simulink model "Water_Tank_Plant_Model"  (R2022b)
settings: Solver=VariableStepAuto  StartTime=0.0  StopTime=inf  RelTol=1e-3
model workspace (MAT data in the model file):
  A = 8
  Boost = 0
  Empty = 0
  Height = 3
  Hin = 8
  Qin = 2
  R = 1
  b = 0
libraries: slpidlib x1
settings Model: Creator=deanlonergan  LastModifiedBy=deanlonergan

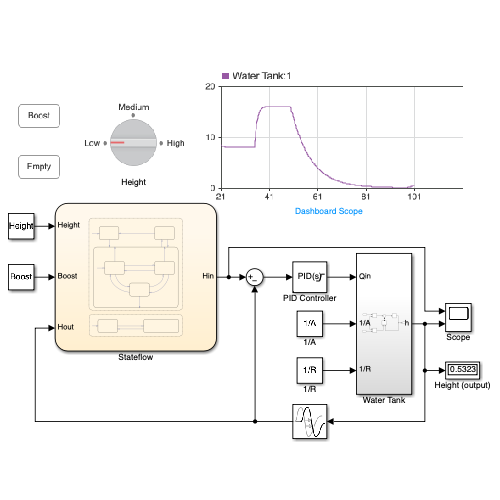
[thumbnail: Simulink's stored preview of the top-level diagram]
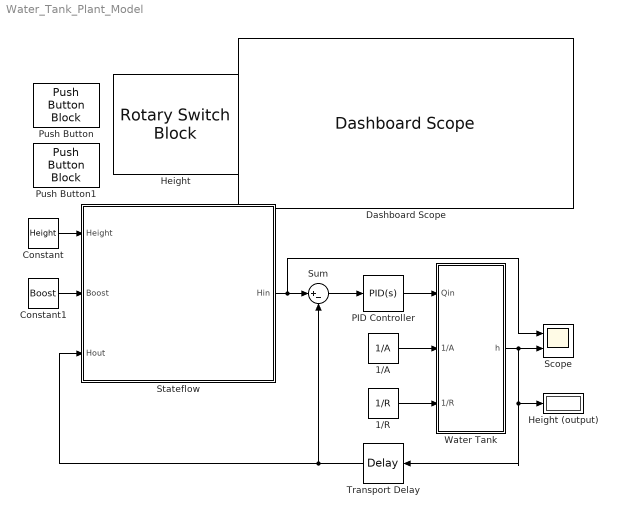
== system Water_Tank_Plant_Model ==
  1/A : Constant  Value=1/A
  1/R : Constant  Value=1/R
  Constant : Constant  Value=Height
  Constant1 : Constant  Value=Boost
  Dashboard Scope : DashboardScope  Ymin=0  Ymax=20  ScaleAtStop=off  UpdateMode=Scroll
  Height : RotarySwitchBlock  LabelPosition=Hide
      settings: Values={{'Low', 'Medium', 'High'}, [1 2 3]}
  Height (output) : Display
  PID Controller : slpidlib/PID Controller  Controller=PID  Form=Parallel  TimeDomain=Continuous-time  UseExternalTs=off  SampleTime=-1  IntegratorMethod=Forward Euler  FilterMethod=Forward Euler  ControllerParametersSource=internal  P=7.2  I=0.92  UseKiTs=on  D=0.29  N=0  UseFilter=on  TunerSelectOption=Transfer Function Based (PID Tuner App)  InitialConditionSource=internal  InitialConditionForIntegrator=0  InitialConditionForFilter=0  DifferentiatorICPrevScaledInput=0  ExternalReset=none  TrackingMode=off  Kt=1  LimitOutput=on  SatLimitsSource=internal  UpperSaturationLimit=50  LowerSaturationLimit=-0  LinearizeAsGain=on  AntiWindupMode=none  Kb=1  LimitIntegrator=off  UpperIntegratorSaturationLimit=inf  LowerIntegratorSaturationLimit=-inf  POutMin=[]  POutMax=[]  IOutMin=[]  IOutMax=[]  DOutMin=[]  DOutMax=[]  NOutMin=[]  NOutMax=[]  SumOutMin=[]  SumOutMax=[]  SaturationOutMin=[]  SaturationOutMax=[]  PParamMin=[]  PParamMax=[]  IParamMin=[]  IParamMax=[]  DParamMin=[]  DParamMax=[]  NParamMin=[]  NParamMax=[]  KbParamMin=[]  KbParamMax=[]  KtParamMin=[]  KtParamMax=[]  KbOutMin=[]  KbOutMax=[]  KtOutMin=[]  KtOutMax=[]  IntegratorOutMin=[]  IntegratorOutMax=[]  FilterOutMin=[]  FilterOutMax=[]  SumI1OutMin=[]  SumI1OutMax=[]  SumI2OutMin=[]  SumI2OutMax=[]  SumI3OutMin=[]  SumI3OutMax=[]  SumI4OutMin=[]  SumI4OutMax=[]  SumDOutMin=[]  SumDOutMax=[]  DifferentiatorOutMin=[]  DifferentiatorOutMax=[]  FilterDiffOutCoefMin=[]  FilterDiffOutCoefMax=[]  ReciprocalOutMin=[]  ReciprocalOutMax=[]  SumDenOutMin=[]  SumDenOutMax=[]  SumNumOutMin=[]  SumNumOutMax=[]  DivideOutMin=[]  DivideOutMax=[]  UdiffTsProdOutMin=[]  UdiffTsProdOutMax=[]  NTsProdOutMin=[]  NTsProdOutMax=[]  UintegralTsProdOutMin=[]  UintegralTsProdOutMax=[]  UngainTsProdOutMin=[]  UngainTsProdOutMax=[]  ClampingZeroOutDataTypeStr=Inherit: Inherit via back propagation  ClampingZeroOutMin=[]  ClampingZeroOutMax=[]  FilterDenConstantOutDataTypeStr=Inherit: Inherit via back propagation  FilterDenConstantOutMin=[]  FilterDenConstantOutMax=[]  PCopyOutDataTypeStr=Inherit: Inherit via back propagation  PCopyOutMin=[]  PCopyOutMax=[]  NCopyOutDataTypeStr=Inherit: Inherit via back propagation  NCopyOutMin=[]  NCopyOutMax=[]  IntegratorContinuousStateAttributes=''  IntegratorStateMustResolveToSignalObject=off  IntegratorRTWStateStorageClass=Auto  FilterContinuousStateAttributes=''  FilterStateMustResolveToSignalObject=off  FilterRTWStateStorageClass=Auto  ParallelPVariant=InternalParameters  IdealPVariant=Disabled  IVariant=InternalParameters  DVariant=InternalParameters  IntegratorVariant=Continuous  SatVariant=Enabled  AWVariant=Passthrough  PCopyVariant=Disabled  TRVariant=Disabled  FdbkBlocksVariant=Forward  IdealPFdbkVariant=Disabled  SatFdbkVariant=Disabled  DerivativeFilterVariant=ContFilter  NVariant=InternalParameters  NCopyVariant=Disabled  FilterICVariant=InternalICsFilter  IntegratorICVariant=InternalICs  ExternalResetVariant=Disabled  TRSumVariant=Passthrough  SumFdbkVariant=Disabled  SumVariant=Sum_PID  TsampFilterVariant=InternalTs  TsampNgainVariant=Passthrough  TsampIntegralVariant=Passthrough  ExternalSaturationOutDataTypeStr=Inherit: Same as second input
  Push Button : PushButtonBlock  ButtonText=Boost  OffValue=0.000000
  Push Button1 : PushButtonBlock  ButtonText=Empty  OnValue=0  OffValue=3.000000
  Scope : Scope  NumInputPorts=2
  Stateflow : Stateflow chart  TreatAsAtomicUnit=on
  Sum : Sum  Inputs=|+-
  Transport Delay : TransportDelay  DelayTime=0.05
  Water Tank : Subsystem
  wires:
  1/A/1 -> Water Tank/2(1/A)
  1/R/1 -> Water Tank/3(1/R)
  Water Tank/1(h) -> Scope/2, Transport Delay/1, Height (output)/1
  Sum/1 -> PID Controller/1
  Stateflow/1(Hin) -> Scope/1, Sum/1
  PID Controller/1 -> Water Tank/1(Qin)
  Transport Delay/1 -> Sum/2, Stateflow/3(Hout)
  Constant/1 -> Stateflow/1(Height)
  Constant1/1 -> Stateflow/2(Boost)

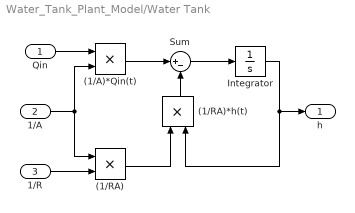
== system Water_Tank_Plant_Model/Water Tank ==
  Qin : Inport
  1/A : Inport  Port=2
  1/R : Inport  Port=3
  (1/A)*Qin(t) : Product
  (1/RA) : Product
  (1/RA)*h(t) : Product
  Integrator : Integrator
  Sum : Sum  Inputs=|+-
  h : Outport
  wires:
  1/A/1 -> (1/RA)/1, (1/A)*Qin(t)/2
  (1/RA)/1 -> (1/RA)*h(t)/1
  Integrator/1 -> h/1, (1/RA)*h(t)/2
  (1/RA)*h(t)/1 -> Sum/2
  Sum/1 -> Integrator/1
  (1/A)*Qin(t)/1 -> Sum/1
  1/R/1 -> (1/RA)/2
  Qin/1 -> (1/A)*Qin(t)/1

== stateflow chart Water_Tank_Plant_Model/Stateflow ==
  state Operating [parallel]
    settings: executionOrder=1
    state Hold
    state Empty
      Hin = 0
    state Fill
      state Low
        Hin = 2
      state High
        Hin = 16
      state Med
        Hin = 8
      Low -> Fill [order 3] : [Height==0]
      High -> Fill [order 3] : [Height==0]
      Low -> High [order 2] : [Height==3]
      (default) -> Low
      High -> Low [order 2] : [Height==1]
      Med -> Low [order 1] : [Height==1]
      Low -> Med [order 1] : [Height==2]
      Med -> High [order 2] : [Height==3]
      High -> Med [order 1] : [Height==2]
      Med -> Fill [order 3] : [Height==0]
    Hold -> Empty [order 2] : [after(5,sec)]
    (default) -> Empty
    Empty -> Fill : [Hout<0.01]
    Fill -> Hold : [Height==0]
    Hold -> Fill [order 1] : [Height>0]
  state Boost [parallel]
    settings: executionOrder=2
    state Off
    state On
      Hin = Hin + (Hin*0.1)
    (default) -> Off
    Off -> On : [Boost==1]
    On -> Off : [after(10,sec)]
  data: Hin output; Height input; Boost input; Hout input
